simulink model "linjar_sim_traj_plan"  (R2022b)
settings: Solver=VariableStepAuto  StartTime=0.0  StopTime=10  RelTol=1e-3
values from neighbouring files (symbols this model uses):
  A = [0    g/2   0    0    0    0    0    0 ... (first row only)    [gain_and_trajectory_calculation.m]
  B = [0          g       0 ... (first row only)    [gain_and_trajectory_calculation.m]
  C = eye(8,8)    [gain_and_trajectory_calculation.m]
undefined symbols (not defined in the file or in its folder): DiscIntNeverNeededParam, K
settings Model: Creator=Edvin  LastModifiedBy=Edvin

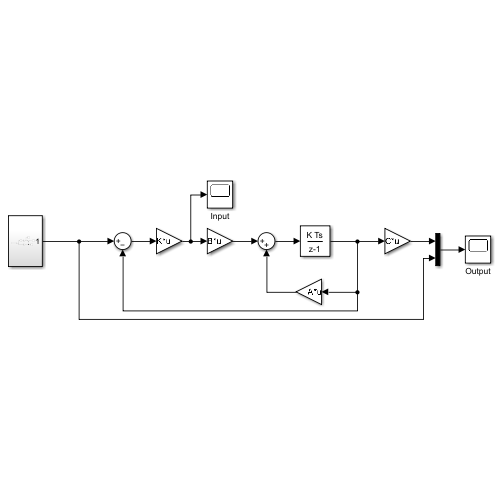
[thumbnail: Simulink's stored preview of the top-level diagram]
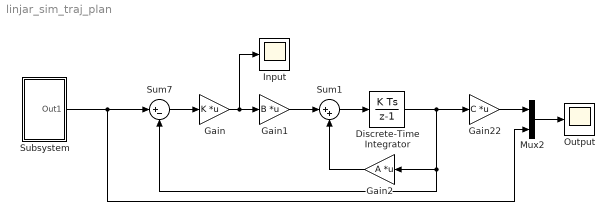
== system linjar_sim_traj_plan ==
  Discrete-Time Integrator : DiscreteIntegrator  SampleTime=-1  ICPrevOutput=DiscIntNeverNeededParam  ICPrevScaledInput=DiscIntNeverNeededParam
  Gain : Gain  Gain=K  Multiplication=Matrix(K*u)
  Gain1 : Gain  Gain=B  Multiplication=Matrix(K*u)
  Gain2 : Gain  Gain=A  Multiplication=Matrix(K*u)
  Gain22 : Gain  Gain=C  Multiplication=Matrix(K*u)
  Input : Scope
  Mux2 : Mux  Inputs=2
  Output : Scope
  Subsystem : Subsystem
  Sum1 : Sum  Inputs=|++
  Sum7 : Sum  Inputs=|+-
  wires:
  Gain22/1 -> Mux2/1
  Discrete-Time Integrator/1 -> Gain22/1, Gain2/1, Sum7/2
  Gain/1 -> Gain1/1, Input/1
  Sum1/1 -> Discrete-Time Integrator/1
  Sum7/1 -> Gain/1
  Gain1/1 -> Sum1/1
  Gain2/1 -> Sum1/2
  Mux2/1 -> Output/1
  Subsystem/1(Out1) -> Mux2/2, Sum7/1

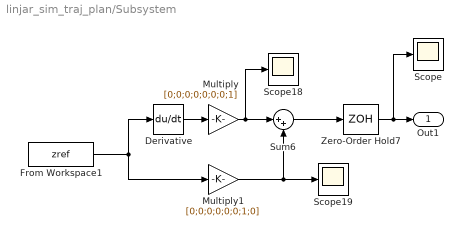
== system linjar_sim_traj_plan/Subsystem ==
  Derivative : Derivative
  From Workspace1 : FromWorkspace  VariableName=zref
  Multiply : Gain  Gain=[0;0;0;0;0;0;0;1]
  Multiply1 : Gain  Gain=[0;0;0;0;0;0;1;0]
  Scope : Scope
  Scope18 : Scope
  Scope19 : Scope
  Sum6 : Sum  Inputs=|++
  Zero-Order Hold7 : ZeroOrderHold  SampleTime=0.01
  Out1 : Outport
  wires:
  Multiply1/1 -> Scope19/1, Sum6/2
  From Workspace1/1 -> Derivative/1, Multiply1/1
  Zero-Order Hold7/1 -> Scope/1, Out1/1
  Multiply/1 -> Scope18/1, Sum6/1
  Derivative/1 -> Multiply/1
  Sum6/1 -> Zero-Order Hold7/1
